simulink library "GFo_Lib_old"  (R2017a)
settings: Solver=VariableStepAuto  StartTime=0.0  StopTime=10.0  RelTol=1e-3
undefined symbols (not defined in the file or in its folder): C_line, Time_Step, VSC01_id0
undefined symbols (not defined in the file): VSC01_Cf, VSC01_Lf, VSC01_Rf
libraries: powerlib x25, Control_Lib x12, simulink x7, powerlib_meascontrol x2
(part 1 of 2)
settings Model: Creator=Frederic_Colas  LastModifiedBy=Frederic_Colas

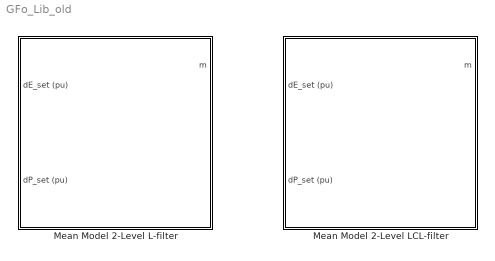
== system GFo_Lib_old ==
  Mean Model 2-Level L-filter : Subsystem  mask(VSC){fn=50, Sn=1000e6, Pn=1000e6, Udcn=640e3, Un1=320e3, Un2=400e3, Rt_pu=0.005, Lt_pu=0.15, Lm_pu=500, Rm_pu=500, Tr_PLL=10e-3, Val_Freq_Support=on, R_percent=4, Rv=0.009, W_TVR=60, I_thresh_pu=1, DX_DR=5, Kp_Rvi_pu=0.676, gainpopup=3, wc1=31.4159, mp1=0.0043, wc2=33.3, mp2=0.0033, wc3=2.5, mp3=0.04, T1=0.1210, T2=0.022, LFpopup=PQ, P0=0.5, Q0=0, V0=1, Theta0=0.57242}
      mask prompts: fn "Nominal Frequency (Hz)"; Sn "Nominal Apparent Power (VA)"; Pn "Nominal Power (W)"; Udcn "Nominal DC Voltage (V)"; Un1 "VSC side Nominal Ph-Ph Voltage (V)"; Un2 "Grid side Nominal Ph-Ph Voltage (V)"; Rt_pu "R (pu)"; Lt_pu "L (pu)"; Lm_pu "Rm (pu)"; Rm_pu "Lm (pu)"; Tr_PLL "Time response (s)"; Val_Freq_Support "Frequency Support"; R_percent "Droop Gain (%)"; Rv "Damping Resistance (Rv)"; W_TVR "Dr filter"; I_thresh_pu "Current Threshold (pu)"; Kp_Rvi_pu "Kp_Rvi"; gainpopup "Strategy"; wc1 "wc"; mp1 "mp"; wc2 "wc"; mp2 "mp"; wc3 "wc"; mp3 "mp"; P0 "Initial Active Power (pu)"; Q0 "Initial Reactive Power (pu)"; V0 "Initial Voltage (pu)"; Theta0 "Initial Angle (°)"
      mask init:
      | % Update Name of LF bus for internal purpose
      |     NameStr = [get_param(gcb,'Name')];% '_LF'];
      |     set_param([gcb '/Load Flow Bus'],'ID',NameStr);    
      |     
      | % Base values
      |     fb = fn;
      |     Pb = Pn;
      |     cos_phi_n = Pn/Sn;
      |     Sb = Pb/cos_phi_n;
      |     Vn1 = Un1/sqrt(3);
      |     Vb1 = Vn1;
      |     Vn2 = Un2/sqrt(3);
      |     Vb2 = Vn2;
      |     Ib1 = Sb / 3*Vb1;
      |     Ib2 = Sb / (3*Vb2);
      |     wb = 2*pi*fb;
      |   
      | % PLL derivation of the parameters
      |     wn_PLL=5/Tr_PLL;
      |     zeta_PLL = 1;
      |     Kp_PLL_pu = 2*zeta_PLL*wn_PLL/wb;
      |     Ki_PLL_pu = wn_PLL^2/wb;
      |     
      | % Set the chosen strategy
      |     Chosen_Strategy = gainpopup;
      |     
      | % Set the frequency droop gain
      |     R = R_percent / 100;
      | 
      | % Compute Initial Voltage of VSC 
      | %   from steady-state output transformer model and Loadflow result
      |     
      |     %Initialize correctly the LoadFlow bus parameters connected to PCC
      |     VLF = V0;
      |     ThetaLF = Theta0;
      |     if (LFpopup == 'PQ')
      |         VLF = 1;
      |         ThetaLF = 0;
      |     elseif (LFpopup == 'PV')
      |         VLF = V0;
      |         ThetaLF = 0;        
      |     end
      |     set_param([gcb '/Load Flow Bus'],'Vref',num2str(VLF),'Vangle',num2str(ThetaLF));
      |     
      |     R1_pu = Rt_pu/2;
      |     L1_pu = Lt_pu/2;
      |     R2_pu = Rt_pu/2;
      |     L2_pu = Lt_pu/2;
      |     X1_pu = L1_pu;
      |     X2_pu = L2_pu;
      |     Xm_pu = Lm_pu;
      |     
      |     Zm_pu = 1/(1/Rm_pu+1/(1i*Xm_pu));
      | 
      |     S0=P0+1i*Q0;
      |     I2 = conj(S0)/(V0);
      | 
      |     Vm = (R2_pu+1i*X2_pu)*I2 + V0;
      |     Im = Vm/Zm_pu;
      | 
      |     I1 = I2 + Im;
      |     V1 = (R1_pu+1i*X1_pu) * I1 + Vm;
      | 
      |     Vvsc0 = abs(V1);
      |     Theta_vsc0 = angle(V1) * 180/pi+Theta0;
      |     
      |     Va0 = Vvsc0*sqrt(2)*Vb1*sin(Theta_vsc0*pi/180);
      |     Vb0 = Vvsc0*sqrt(2)*Vb1*sin(Theta_vsc0*pi/180-2*pi/3);
      |     Vc0 = Vvsc0*sqrt(2)*Vb1*sin(Theta_vsc0*pi/180+2*pi/3);
      |     
      | % Generate string to display LF results on Mask
      |     %str_tmp = fprintf("Vvsc0 = %d, Theta_vsc0 = %d°",Vvsc0,Theta_vsc0);
      |     mo = get_param(gcb,'MaskObject');
      |     mo.getDialogControl('LF_vsc_str').Prompt = ['V0 = ', num2str(Vvsc0),' pu, Angle = ', num2str(Theta_vsc0),'°'];
      |     mo.getDialogControl('LF_pcc_str').Prompt = ['V0 = ', num2str(V0),' pu, Angle = ', num2str(Theta0),'°'];
      |     mo.getDialogControl('LF_pcc_Power_str').Prompt = ['P0 = ', num2str(P0),' pu, Q0 = ', num2str(Q0),' pu'];
      |     %set_param([gcb],'LF_str',str_tmp);
      settings: OpenFcn=|
      | NameStr = get_param(gcb,'Name');
      | open_system(gcbh, 'Mask');
      | 
      | h2AllOpenDlgs = DAStudio.ToolRoot.getOpenDialogs;
      | 
      | for i=1:length(h2AllOpenDlgs)
      |     try
      |          %disp(h2AllOpenDlgs(i).getSource.getBlock.Name);
      |         Dialog_block_name = h2AllOpenDlgs(i).getSource.getBlock.Name;
      |          %strcmp(Dialog_block_name, NameStr),
      |         if (strcmp(h2AllOpenDlgs(i).getSource.getBlock.Name, NameStr))
      |             iPos = h2AllOpenDlgs(i).position;
      |             h2AllOpenDlgs(i).position = [iPos(1)   iPos(2)   iPos(3)*1.4   iPos(4)];
      |         end
      |     end
      | end
      mask TypeOptions gainpopup: 1 | 2 | 3
      mask Callback gainpopup:
      | % Get the mask parameter values. This is a cell
      | %   array of character vectors.
      | maskStr = get_param(gcb,'gainpopup');
      | p=Simulink.Mask.get(gcb);
      | 
      | % The pop-up menu is the first mask parameter.
      | %   Check the value selected in the pop-up
      | if strcmp(maskStr,'1'),
      | 
      |     % Set the visibility of both parameters on when
      |     %   User-defined is selected in the pop-up.
      |     p.getDialogControl('Param_Strat_1').Visible='on';
      |     p.getDialogControl('Param_Strat_2').Visible='off';
      |     p.getDialogControl('Param_Strat_3').Visible='off';
      | 
      | elseif strcmp(maskStr,'2'),
      | 
      |     % Set the visibility of both parameters on when
      |     %   User-defined is selected in the pop-up.
      |     p.getDialogControl('Param_Strat_1').Visible='off';
      |     p.getDialogControl('Param_Strat_2').Visible='on';
      |     p.getDialogControl('Param_Strat_3').Visible='off';
      | 
      |     % Turn off the visibility of the Value field
      |     %   when User-defined is not selected.
      | else
      | 
      |     % Set the visibility of both parameters on when
      |     %   User-defined is selected in the pop-up.
      |     p.getDialogControl('Param_Strat_1').Visible='off';
      |     p.getDialogControl('Param_Strat_2').Visible='off';
      |     p.getDialogControl('Param_Strat_3').Visible='on';
      | 
      | end
      mask TypeOptions LFpopup: Swing | PQ | PV
      mask Callback LFpopup:
      | % Get the mask parameter values. This is a cell
      | %   array of character vectors.
      | maskStr = get_param(gcb,'LFpopup');
      | p=Simulink.Mask.get(gcb);
      | 
      | % The pop-up menu is the first mask parameter.
      | %   Check the value selected in the pop-up
      | if strcmp(maskStr,'Swing'),
      | 
      |     % Set the visibility of both parameters on when
      |     %   User-defined is selected in the pop-up.
      |     p.getParameter('P0').Visible='off';
      |     p.getParameter('Q0').Visible='off';
      |     p.getParameter('V0').Visible='on';
      |     p.getParameter('Theta0').Visible='on';
      |     set_param([gcb '/Source_For_LF'],'BusType','swing');
      | 
      | elseif strcmp(maskStr,'PQ'),
      | 
      |     % Set the visibility of both parameters on when
      |     %   User-defined is selected in the pop-up.
      |     p.getParameter('P0').Visible='on';
      |     p.getParameter('Q0').Visible='on';
      |     p.getParameter('V0').Visible='off';
      |     p.getParameter('Theta0').Visible='off';
      |     set_param([gcb '/Source_For_LF'],'BusType','PQ');
      | 
      |     % Turn off the visibility of the Value field
      |     %   when User-defined is not selected.
      | else
      | 
      |     % Set the visibility of both parameters on when
      |     %   User-defined is selected in the pop-up.
      |     p.getParameter('P0').Visible='on';
      |     p.getParameter('Q0').Visible='off';
      |     p.getParameter('V0').Visible='on';
      |     p.getParameter('Theta0').Visible='off';
      |     set_param([gcb '/Source_For_LF'],'BusType','PV');
      | 
      | end
      mask DialogControl Title_Strat_1 Prompt: Strategy 1
      mask DialogControl Title_Strat_2 Prompt: Strategy 2
      mask DialogControl Title_Strat_3 Prompt: Strategy 3
      mask DialogControl Control4 Prompt: Initial Operating Point
      mask DialogControl Container24 Prompt: VSC side
      mask DialogControl LF_vsc_str Prompt: V0 = 1.0055 pu, Angle = 4.8589°
      mask DialogControl Container25 Prompt: PCC
      mask DialogControl UpdateLoadflow Prompt: Update Loadflow
      mask DialogControl UpdateLoadflow Callback: LoadFlow_VSC
      mask Display:
      | disp('L-Filter');
      | port_label('input',1,'dE_set (pu)');
      | port_label('input',2,'dP_set (pu)');
      | port_label('output',1,'m');
      | port_label('rconn',1,'A');
      | port_label('rconn',2,'B');
      | port_label('rconn',3,'C');
  Mean Model 2-Level LCL-filter : Subsystem  mask(VSC){fn=50, Sn=1000e6, Pn=1000e6, Udcn=640e3, Un1=320e3, Un2=400e3, Rt_pu=0.005, Lt_pu=0.15, Rm_pu=500, Lm_pu=500, Lf_pu=0.15, Rf_pu=0.005, Cf_pu=0.066, Tr_PLL=10e-3, Val_Freq_Support=on, Val_gamma=on, R_percent=4, Rv=0.009, W_TVR=60, I_thresh_pu=1, DX_DR=5, Kp_Rvi_pu=0.676, gainpopup=3, wc1=31.4159, mp1=0.0043, wc2=33.3, mp2=0.0033, wc3=2.5, mp3=0.04, T1=0.1210, T2=0.022, LFpopup=PV, P0=0.1, Q0=0, V0=1, Theta0=13.5501, innercontrol=1, Kp_i=0.73, Ki_i=1.19, Kp_v=0.52, Ki_v=1.16, Kffv=1, Kffi=1, I_max=1.25}
      mask prompts: fn "Nominal Frequency (Hz)"; Sn "Nominal Apparent Power (VA)"; Pn "Nominal Power (W)"; Udcn "Nominal DC Voltage (V)"; Un1 "VSC side Nominal Ph-Ph Voltage (V)"; Un2 "Grid side Nominal Ph-Ph Voltage (V)"; Rt_pu "R (pu)"; Lt_pu "L (pu)"; Rm_pu "Rm (pu)"; Lm_pu "Lm (pu)"; Lf_pu "Lf (pu)"; Rf_pu "Rf (pu)"; Cf_pu "Cf (pu)"; Tr_PLL "Time response (s)"; Val_Freq_Support "Frequency Support"; Val_gamma "gamma activation"; R_percent "Droop Gain (%)"; Rv "Damping Resistance (Rv)"; W_TVR "Dr filter"; I_thresh_pu "Current Threshold (pu)"; Kp_Rvi_pu "Kp_Rvi"; gainpopup "Strategy"; wc1 "wc"; mp1 "mp"; wc2 "wc"; mp2 "mp"; wc3 "wc"; mp3 "mp"; P0 "Initial Active Power (pu)"; Q0 "Initial Reactive Power (pu)"; V0 "Initial Voltage (pu)"; Theta0 "Initial Angle (°)"; innercontrol "Strategy"
      mask init:
      | % Update Name of LF bus for internal purpose
      |     NameStr = [get_param(gcb,'Name')];% '_LF'];
      |     set_param([gcb '/Load Flow Bus'],'ID',NameStr);
      |     %disp(NameStr);
      | 
      | % Base values
      |     % 1 = VSC side
      |     % 2 = grid side
      |     fb = fn;
      |     Pb = Pn;
      |     cos_phi_n = Pn/Sn;
      |     Sb = Pb/cos_phi_n;
      |     Vn1 = Un1/sqrt(3);
      |     Vb1 = Vn1;
      |     Vn2 = Un2/sqrt(3);
      |     Vb2 = Vn2;
      |     Ib1 = Sb / (3*Vb1);
      |     Ib2 = Sb / (3*Vb2);
      |     Zb = (3*Vb1^2)/Sb;
      |     wb = 2*pi*fb;  wb_pu=1;
      |     Lb = Zb/wb;
      |     Cb = 1/(Zb*wb);
      |   
      | % PLL derivation of the parameters
      |     wn_PLL=5/Tr_PLL;
      |     zeta_PLL = 1;
      |     Kp_PLL_pu = 2*zeta_PLL*wn_PLL/wb;
      |     Ki_PLL_pu = wn_PLL^2/wb;
      |     
      | % Set the chosen strategy
      |     Chosen_Strategy = gainpopup;
      |     
      | % Set the frequency droop gain
      |     R = R_percent/100;
      | 
      | % Compute Initial Voltage of VSC 
      | %   from steady-state output transformer model and Loadflow result
      |     
      |     %Initialize correctly the LoadFlow bus parameters connected to PCC
      |     VLF = V0;
      |     ThetaLF = Theta0;
      |     if (LFpopup == 'PQ')
      |         VLF = 1;
      |         ThetaLF = 0;
      |     elseif (LFpopup == 'PV')
      |         VLF = V0;
      |         ThetaLF = 0;        
      |     end
      |     set_param([gcb '/Load Flow Bus'],'Vref',num2str(VLF),'Vangle',num2str(ThetaLF));
      | 
      |     % steady-state model of output transformer
      |     Rf_pu = Rt_pu;
      |     R1_pu = Rt_pu/2;
      |     L1_pu = Lt_pu/2;
      |     R2_pu = Rt_pu/2;
      |     L2_pu = Lt_pu/2;
      |     X1_pu = L1_pu;
      |     X2_pu = L2_pu;
      |     Xm_pu = Lm_pu;
      |     wb_pu = 1;
      |     
      |     Zm_pu = 1/(1/Rm_pu+1/(1i*Xm_pu));
      |     S0=P0+1i*Q0;
      |     I2 = conj(S0)/(V0);
      |     Vm = (R2_pu+1i*X2_pu)*I2 + V0;
      |     Im = Vm/Zm_pu;
      |     I1 = I2 + Im;
      |     V1 = (R1_pu+1i*X1_pu) * I1 + Vm;
      |     
      |     Eg0 = abs(V1); % compute initial Eg value
      |     Theta_m0 = angle(V1) * 180/pi+Theta0;
      |     
      |     %Steady-state model of LC Filter
      |     Is = I1 + 1i*Cf_pu*V1;
      |     Theta_Is = angle(Is) * 180/pi+Theta0;
      |     Vm = (1i*Lf_pu+Rf_pu)*Is+ V1;  %  
      |     
      | % Generate string to display LF results on Mask
      |     %str_tmp = fprintf("Vvsc0 = %d, Theta_vsc0 = %d°",Vvsc0,Theta_vsc0);
      |     mo = get_param(gcb,'MaskObject');
      |     mo.getDialogControl('LF_pcc_str').Prompt = ['V0 = ', num2str(V0),' pu, Angle = ', num2str(Theta0),'°'];
      |     mo.getDialogControl('LF_pcc_Power_str').Prompt = ['P0 = ', num2str(P0),' pu, Q0 = ', num2str(Q0),' pu'];
      |     %set_param([gcb],'LF_str',str_tmp);
      |  %GRD00_Theta0 = Theta0;
      |  % Initial current and voltage states calculation 
      |  
      | % Given Setpoint in PV bus
      |  
      | Vg0_d=V0*cos(Theta0*pi/180-Theta_m0*pi/180);
      | Vg0_q=V0*sin(Theta0*pi/180-Theta_m0*pi/180);
      | Vg0_dq = [Vg0_d ;Vg0_q; 0];
      |  
      | % Initial state of AC grid current : Ig0dq
      | 
      | Theta_I2 = angle(I2) * 180/pi + Theta0;
      | Ig0_d = abs(I2)*cos(Theta_I2*pi/180-Theta_m0*pi/180);
      | Ig0_q = abs(I2)*sin(Theta_I2*pi/180-Theta_m0*pi/180);
      | Ig0_dq = [Ig0_d; Ig0_q; 0];
      |  
      | % Initial state of capacitor voltage : eg0dq
      | 
      | Eg0_d = Eg0;
      | Eg0_q = 0;
      | Eg0_dq = [Eg0; 0; 0];
      |  
      | % Initial state of VSC Current : Is0dq
      | 
      | Is0_d = abs(Is) * cos(Theta_Is*pi/180-Theta_m0*pi/180);
      | Is0_q = abs(Is) * sin(Theta_Is*pi/180-Theta_m0*pi/180);
      | Is0_dq = [Is0_d; Is0_q; 0];
      | 
      | % Initial state of Modulation Voltage : Vm0dq
      | 
      | Vvsc0 = abs(Vm);
      | Theta_vsc0 = angle(Vm)*180/pi + Theta0;
      | Vm0_d = Vvsc0 * cos(Theta_vsc0*pi/180-Theta_m0*pi/180);
      | Vm0_q = Vvsc0 * sin(Theta_vsc0*pi/180-Theta_m0*pi/180);
      |  
      | Va0 = sqrt(2)*Vb1*Vvsc0*sin(Theta_vsc0*pi/180);
      | Vb0 = sqrt(2)*Vb1*Vvsc0*sin(Theta_vsc0*pi/180-2*pi/3);
      | Vc0 = sqrt(2)*Vb1*Vvsc0*sin(Theta_vsc0*pi/180+2*pi/3);
      | Vabc0 = [Va0 Vb0 Vc0];
      |  
      | mo.getDialogControl('LF_vsc_str').Prompt = ['V0 = ', num2str(Eg0),' pu, Angle = ', num2str(Theta_m0),'°'];
      settings: OpenFcn=|
      | NameStr = get_param(gcb,'Name');
      | open_system(gcbh, 'Mask');
      | 
      | h2AllOpenDlgs = DAStudio.ToolRoot.getOpenDialogs;
      | 
      | for i=1:length(h2AllOpenDlgs)
      |     try
      |          %disp(h2AllOpenDlgs(i).getSource.getBlock.Name);
      |         Dialog_block_name = h2AllOpenDlgs(i).getSource.getBlock.Name;
      |          %strcmp(Dialog_block_name, NameStr),
      |         if (strcmp(h2AllOpenDlgs(i).getSource.getBlock.Name, NameStr))
      |             iPos = h2AllOpenDlgs(i).position;
      |             h2AllOpenDlgs(i).position = [iPos(1)   iPos(2)   iPos(3)*1.6   iPos(4)];
      |         end
      |     end
      | end
      mask TypeOptions gainpopup: 1 | 2 | 3
      mask Callback gainpopup:
      | % Get the mask parameter values. This is a cell
      | %   array of character vectors.
      | maskStr = get_param(gcb,'gainpopup');
      | p=Simulink.Mask.get(gcb);
      | 
      | % The pop-up menu is the first mask parameter.
      | %   Check the value selected in the pop-up
      | if strcmp(maskStr,'1'),
      | 
      |     % Set the visibility of both parameters on when
      |     %   User-defined is selected in the pop-up.
      |     p.getDialogControl('Param_Strat_1').Visible='on';
      |     p.getDialogControl('Param_Strat_2').Visible='off';
      |     p.getDialogControl('Param_Strat_3').Visible='off';
      | 
      | 
      | elseif strcmp(maskStr,'2'),
      | 
      |     % Set the visibility of both parameters on when
      |     %   User-defined is selected in the pop-up.
      |     p.getDialogControl('Param_Strat_1').Visible='off';
      |     p.getDialogControl('Param_Strat_2').Visible='on';
      |     p.getDialogControl('Param_Strat_3').Visible='off';
      | 
      | 
      |     % Turn off the visibility of the Value field
      |     %   when User-defined is not selected.
      | elseif strcmp(maskStr,'3'),
      | 
      |     % Set the visibility of both parameters on when
      |     %   User-defined is selected in the pop-up.
      |     p.getDialogControl('Param_Strat_1').Visible='off';
      |     p.getDialogControl('Param_Strat_2').Visible='off';
      |     p.getDialogControl('Param_Strat_3').Visible='on';
      | 
      | else
      | 
      |     % Set the visibility of both parameters on when
      |     %   User-defined is selected in the pop-up.
      |     p.getDialogControl('Param_Strat_1').Visible='off';
      |     p.getDialogControl('Param_Strat_2').Visible='off';
      |     p.getDialogControl('Param_Strat_3').Visible='off';
      | 
      | end
      mask TypeOptions LFpopup: Swing | PQ | PV
      mask Callback LFpopup:
      | % Get the mask parameter values. This is a cell
      | %   array of character vectors.
      | maskStr = get_param(gcb,'LFpopup');
      | p=Simulink.Mask.get(gcb);
      | 
      | % The pop-up menu is the first mask parameter.
      | %   Check the value selected in the pop-up
      | if strcmp(maskStr,'Swing'),
      | 
      |     % Set the visibility of both parameters on when
      |     %   User-defined is selected in the pop-up.
      |     p.getParameter('P0').Visible='off';
      |     p.getParameter('Q0').Visible='off';
      |     p.getParameter('V0').Visible='on';
      |     p.getParameter('Theta0').Visible='on';
      |     set_param([gcb '/Source_For_LF'],'BusType','swing');
      | 
      | elseif strcmp(maskStr,'PQ'),
      | 
      |     % Set the visibility of both parameters on when
      |     %   User-defined is selected in the pop-up.
      |     p.getParameter('P0').Visible='on';
      |     p.getParameter('Q0').Visible='on';
      |     %p.getParameter('V0').Value='1';
      |     %set_param(gcb,'V0','1');
      |     p.getParameter('V0').Visible='off';
      |     p.getParameter('Theta0').Visible='off';
      |     set_param([gcb '/Source_For_LF'],'BusType','PQ');
      | 
      |     % Turn off the visibility of the Value field
      |     %   when User-defined is not selected.
      | else
      | 
      |     % Set the visibility of both parameters on when
      |     %   User-defined is selected in the pop-up.
      |     p.getParameter('P0').Visible='on';
      |     p.getParameter('Q0').Visible='off';
      |     p.getParameter('V0').Visible='on';
      |     p.getParameter('Theta0').Visible='off';
      |     set_param([gcb '/Source_For_LF'],'BusType','PV');
      | 
      | end
      mask TypeOptions innercontrol: 1
      mask Callback innercontrol:
      | % Get the mask parameter values. This is a cell
      | %   array of character vectors.
      | maskStr = get_param(gcb,'innercontrol');
      | p=Simulink.Mask.get(gcb);
      | 
      | % The pop-up menu is the first mask parameter.
      | %   Check the value selected in the pop-up
      | if strcmp(maskStr,'1'),
      | 
      |     % Set the visibility of both parameters on when
      |     %   User-defined is selected in the pop-up.
      |     p.getDialogControl('Param_Strat_11').Visible='on';
      | 
      | 
      | else
      | 
      |     % Set the visibility of both parameters on when
      |     %   User-defined is selected in the pop-up.
      |     p.getDialogControl('Param_Strat_11').Visible='on';
      | 
      | end
      mask DialogControl Title_Strat_1 Prompt: Strategy 1
      mask DialogControl Title_Strat_2 Prompt: Strategy 2
      mask DialogControl Title_Strat_3 Prompt: Strategy 3
      mask DialogControl Control4 Prompt: Initial Operating Point
      mask DialogControl Container24 Prompt: VSC side
      mask DialogControl LF_vsc_str Prompt: V0 = 1.0008 pu, Angle = 14.4173°
      mask DialogControl Container25 Prompt: PCC
      mask DialogControl UpdateLoadflow Prompt: Update Loadflow
      mask DialogControl UpdateLoadflow Callback: LoadFlow_VSC
      mask DialogControl Title_Strat_11 Prompt: Cascaded_control
      mask Display:
      | disp('LCL-Filter');
      | port_label('input',1,'dE_set (pu)');
      | port_label('input',2,'dP_set (pu)');
      | port_label('output',1,'m');
      | port_label('rconn',1,'A');
      | port_label('rconn',2,'B');
      | port_label('rconn',3,'C');

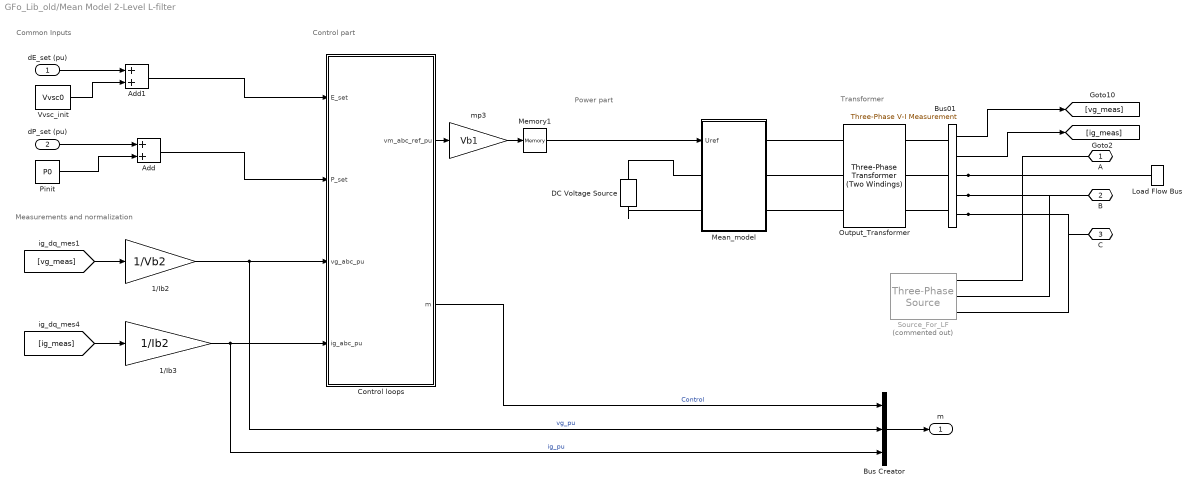
== system GFo_Lib_old/Mean Model 2-Level L-filter ==
  note: Control part
  note: Measurements and normalization
  note: Power part
  note: Common Inputs
  note: Transformer
  dE_set (pu) : Inport
  dP_set (pu) : Inport  Port=2
  1/Ib2 : Gain  Gain=1/Vb2
  1/Ib3 : Gain  Gain=1/Ib2
  Add : Sum
  Add1 : Sum
  Bus Creator : BusCreator  Inputs=3
  Bus01 : powerlib/Measurements/Three-Phase V-I Measurement  VoltageMeasurement=phase-to-ground  SetLabelV=off  LabelV=Vabc  Vpu=off  VpuLL=off  CurrentMeasurement=yes  SetLabelI=off  LabelI=Iabc  Ipu=off  Pbase=100e6  Vbase=500e3  OutputType=Complex  PhasorSimulation=off  PSBequivalent=0
  Control loops : Subsystem
  DC Voltage Source : powerlib/Electrical Sources/DC Voltage Source  Amplitude=Udcn  Measurements=Voltage
  Load Flow Bus : powerlib/Measurements/Load Flow Bus  LConnTagsString=a  Phases=single  Connectors=on one side  ID=Mean Model 2-Level L-filter  Vbase=Un2  Vref=1  Vangle=0.57242  VLF=1.001  VLFb=1  VLFc=1  angleLF=0.5724  angleLFb=0  angleLFc=0
      settings: SourceProductName=Simscape Power Systems
  Mean_model : Subsystem
  Memory1 : Memory  X0=[Va0 Vb0 Vc0]
  Output_Transformer : powerlib/Elements/Three-Phase Transformer (Two Windings)  Winding1Connection=Yg  Winding2Connection=Yg  CoreType=Three single-phase transformers  SetSaturation=off  Hysteresis=off  DataFile='hysteresis'  SetInitialFlux=off  Measurements=None  UNITS=pu  NominalPower=[Sn , fb]  Winding1=[Un1 , Rt_pu/2 , Lt_pu/2]  Winding2=[Un2 , Rt_pu/2 , Lt_pu/2]  Rm=Rm_pu  Lm=Lm_pu  L0=0.5  Saturation=[ 0,0 ; 0.0024,1.2 ; 1.0,1.52 ]  InitialFluxes=[ 0.8 , -0.8 , 0.7 ]  MoreParameters=off  BreakLoop=off  DataType=off  TransfoNumber=1
  Pinit : Constant  Value=P0
  Source_For_LF : powerlib/Electrical Sources/Three-Phase Source  Commented=on  InternalConnection=Yg  VoltagePhases=off  Voltage=Un2  PhaseAngle=0  Voltage_phases=[25e3 25e3 25e3]/sqrt(3)  PhaseAngles_phases=[0 -120 +120]  Frequency=fb  NonIdealSource=off  SpecifyImpedance=off  Resistance=0  Inductance=0  ShortCircuitLevel=100e6  BaseVoltage=Un  XRratio=7  BusType=PQ  Pref=P0*Sb  Qref=Q0*Sb  Prefabc=[10e3, 10e3, 10e3]  Qrefabc=[0, 0, 0]  Qmin=-inf  Qmax=inf
  Vvsc_init : Constant  Value=Vvsc0
  mp3 : Gain  Gain=Vb1
  A : PMIOPort  Port=1  Side=Right
  B : PMIOPort  Port=2  Side=Right
  C : PMIOPort  Port=3  Side=Right
  m : Outport
  wires:
  [ig_meas] -> 1/Ib3/1
  Bus01/2 -> [ig_meas]
  dE_set (pu)/1 -> Add1/1
  Bus01/1 -> [vg_meas]
  Vvsc_init/1 -> Add1/2
  Pinit/1 -> Add/2
  dP_set (pu)/1 -> Add/1
  Memory1/1 -> Mean_model/1(Uref)
  Add1/1 -> Control loops/1(E_set)
  Control loops/1(vm_abc_ref_pu) -> mp3/1
  [vg_meas] -> 1/Ib2/1
  Bus Creator/1 -> m/1
  1/Ib2/1 -> Control loops/3(vg_abc_pu), Bus Creator/2  "vg_pu"
  1/Ib3/1 -> Control loops/4(ig_abc_pu), Bus Creator/3  "ig_pu"
  mp3/1 -> Memory1/1
  Control loops/2(m) -> Bus Creator/1  "Control"
  Add/1 -> Control loops/2(P_set)
  connections:
  Bus01/RConn3 -- C/RConn1 -- Source_For_LF/RConn3
  Bus01/RConn1 -- A/RConn1 -- Load Flow Bus/LConn1 -- Source_For_LF/RConn1
  Mean_model/RConn3 -- Output_Transformer/LConn3
  Mean_model/RConn2 -- Output_Transformer/LConn2
  Mean_model/RConn1 -- Output_Transformer/LConn1
  Bus01/RConn2 -- B/RConn1 -- Source_For_LF/RConn2
  Output_Transformer/RConn3 -- Bus01/LConn3
  DC Voltage Source/RConn1 -- Mean_model/LConn1
  Output_Transformer/RConn2 -- Bus01/LConn2
  Output_Transformer/RConn1 -- Bus01/LConn1
  DC Voltage Source/LConn1 -- Mean_model/LConn2

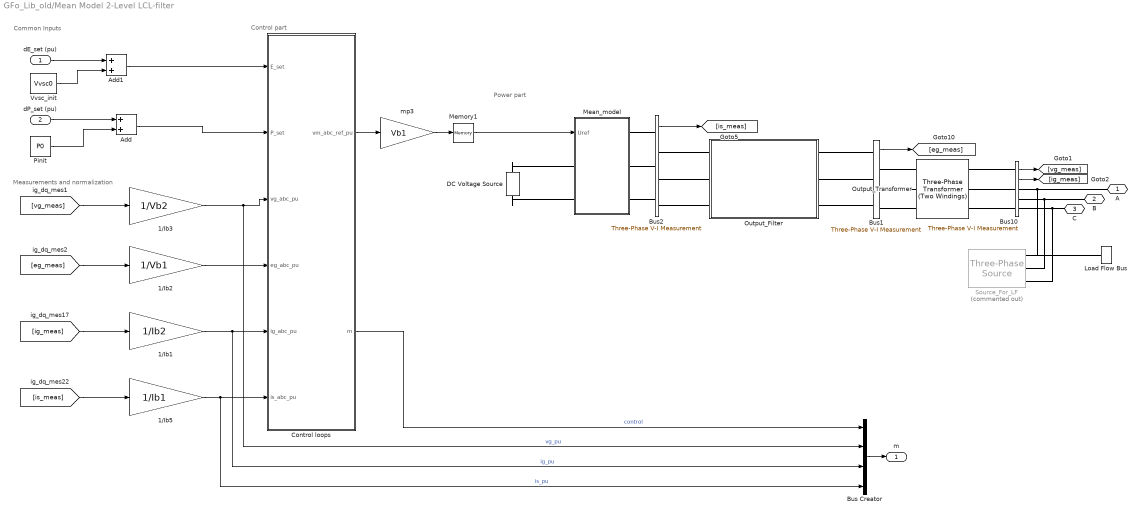
== system GFo_Lib_old/Mean Model 2-Level LCL-filter ==
  note: Control part
  note: Measurements and normalization
  note: Power part
  note: Common Inputs
  dE_set (pu) : Inport
  dP_set (pu) : Inport  Port=2
  1/Ib1 : Gain  Gain=1/Ib2
  1/Ib2 : Gain  Gain=1/Vb1
  1/Ib3 : Gain  Gain=1/Vb2
  1/Ib5 : Gain  Gain=1/Ib1
  Add : Sum
  Add1 : Sum
  Bus Creator : BusCreator  Inputs=4
  Bus1 : powerlib/Measurements/Three-Phase V-I Measurement  VoltageMeasurement=phase-to-ground  SetLabelV=off  LabelV=Vabc  Vpu=off  VpuLL=off  CurrentMeasurement=no  SetLabelI=off  LabelI=Iabc  Ipu=off  Pbase=100e6  Vbase=500e3  OutputType=Complex  PhasorSimulation=off  PSBequivalent=0
  Bus10 : powerlib/Measurements/Three-Phase V-I Measurement  VoltageMeasurement=phase-to-ground  SetLabelV=off  LabelV=Vabc  Vpu=off  VpuLL=off  CurrentMeasurement=yes  SetLabelI=off  LabelI=Iabc  Ipu=off  Pbase=100e6  Vbase=500e3  OutputType=Complex  PhasorSimulation=off  PSBequivalent=0
  Bus2 : powerlib/Measurements/Three-Phase V-I Measurement  VoltageMeasurement=no  SetLabelV=off  LabelV=Vabc  Vpu=off  VpuLL=off  CurrentMeasurement=yes  SetLabelI=off  LabelI=Iabc  Ipu=off  Pbase=100e6  Vbase=500e3  OutputType=Complex  PhasorSimulation=off  PSBequivalent=0
  Control loops : Subsystem
  DC Voltage Source : powerlib/Electrical Sources/DC Voltage Source  Amplitude=Udcn  Measurements=Voltage
  Load Flow Bus : powerlib/Measurements/Load Flow Bus  LConnTagsString=a  Phases=single  Connectors=on one side  ID=Mean Model 2-Level LCL-filter  Vbase=Un2  Vref=1  Vangle=13.5501  VLF=0.9956  VLFb=1  VLFc=1  angleLF=13.55  angleLFb=0  angleLFc=0
      settings: SourceProductName=Simscape Power Systems
  Mean_model : Subsystem
  Memory1 : Memory  X0=[Va0 Vb0 Vc0]
  Output_Filter : Subsystem  mask{Lf=VSC01_Lf, Rf=VSC01_Rf, Cf=VSC01_Cf}
      mask prompts: Lf "Filter inductance [H]"; Rf "Filter resistance [R]"; Cf "Filter capacitance [F]"
  Output_Transformer : powerlib/Elements/Three-Phase Transformer (Two Windings)  Winding1Connection=Yg  Winding2Connection=Yg  CoreType=Three single-phase transformers  SetSaturation=off  Hysteresis=off  DataFile='hysteresis'  SetInitialFlux=off  Measurements=None  UNITS=pu  NominalPower=[Sn , fb]  Winding1=[Un1 , Rt_pu/2 , Lt_pu/2]  Winding2=[Un2 , Rt_pu/2 , Lt_pu/2]  Rm=Rm_pu  Lm=Lm_pu  L0=0.5  Saturation=[ 0,0 ; 0.0024,1.2 ; 1.0,1.52 ]  InitialFluxes=[-1.0109960716468 0.506091473811006 0.504904597835851]  MoreParameters=off  BreakLoop=off  DataType=off  TransfoNumber=1
  Pinit : Constant  Value=P0
  Source_For_LF : powerlib/Electrical Sources/Three-Phase Source  Commented=on  InternalConnection=Yg  VoltagePhases=off  Voltage=Un2*V0  PhaseAngle=Theta0  Voltage_phases=[25e3 25e3 25e3]/sqrt(3)  PhaseAngles_phases=[0 -120 +120]  Frequency=fb  NonIdealSource=off  SpecifyImpedance=off  Resistance=0  Inductance=0  ShortCircuitLevel=100e6  BaseVoltage=Un  XRratio=7  BusType=PV  Pref=P0*Sb  Qref=Q0*Sb  Prefabc=[10e3, 10e3, 10e3]  Qrefabc=[0, 0, 0]  Qmin=-inf  Qmax=inf
  Vvsc_init : Constant  Value=Vvsc0
  mp3 : Gain  Gain=Vb1
  A : PMIOPort  Port=1  Side=Right
  B : PMIOPort  Port=2  Side=Right
  C : PMIOPort  Port=3  Side=Right
  m : Outport
  wires:
  Add/1 -> Control loops/2(P_set)
  dE_set (pu)/1 -> Add1/1
  Bus1/1 -> [eg_meas]
  Add1/1 -> Control loops/1(E_set)
  Vvsc_init/1 -> Add1/2
  Pinit/1 -> Add/2
  dP_set (pu)/1 -> Add/1
  Bus10/1 -> [vg_meas]
  Bus2/1 -> [is_meas]
  mp3/1 -> Memory1/1
  Bus10/2 -> [ig_meas]
  1/Ib1/1 -> Control loops/5(ig_abc_pu), Bus Creator/3  "ig_pu"
  1/Ib3/1 -> Bus Creator/2, Control loops/3(vg_abc_pu)  "vg_pu"
  Control loops/2(m) -> Bus Creator/1  "control"
  Bus Creator/1 -> m/1
  1/Ib2/1 -> Control loops/4(eg_abc_pu)
  1/Ib5/1 -> Control loops/6(is_abc_pu), Bus Creator/4  "is_pu"
  Control loops/1(vm_abc_ref_pu) -> mp3/1
  Memory1/1 -> Mean_model/1(Uref)
  [vg_meas] -> 1/Ib3/1
  [eg_meas] -> 1/Ib2/1
  [ig_meas] -> 1/Ib1/1
  [is_meas] -> 1/Ib5/1
  connections:
  DC Voltage Source/RConn1 -- Mean_model/LConn1
  DC Voltage Source/LConn1 -- Mean_model/LConn2
  Bus1/LConn1 -- Output_Filter/RConn1
  Bus1/LConn2 -- Output_Filter/RConn2
  Bus1/LConn3 -- Output_Filter/RConn3
  Output_Transformer/LConn1 -- Bus1/RConn1
  Bus1/RConn2 -- Output_Transformer/LConn2
  Bus1/RConn3 -- Output_Transformer/LConn3
  Bus10/LConn1 -- Output_Transformer/RConn1
  Bus10/LConn2 -- Output_Transformer/RConn2
  Bus10/LConn3 -- Output_Transformer/RConn3
  C/RConn1 -- Source_For_LF/RConn3 -- Bus10/RConn3
  B/RConn1 -- Source_For_LF/RConn2 -- Bus10/RConn2
  A/RConn1 -- Load Flow Bus/LConn1 -- Source_For_LF/RConn1 -- Bus10/RConn1
  Bus2/LConn1 -- Mean_model/RConn1
  Bus2/LConn2 -- Mean_model/RConn2
  Bus2/LConn3 -- Mean_model/RConn3
  Bus2/RConn1 -- Output_Filter/LConn1
  Bus2/RConn2 -- Output_Filter/LConn2
  Bus2/RConn3 -- Output_Filter/LConn3

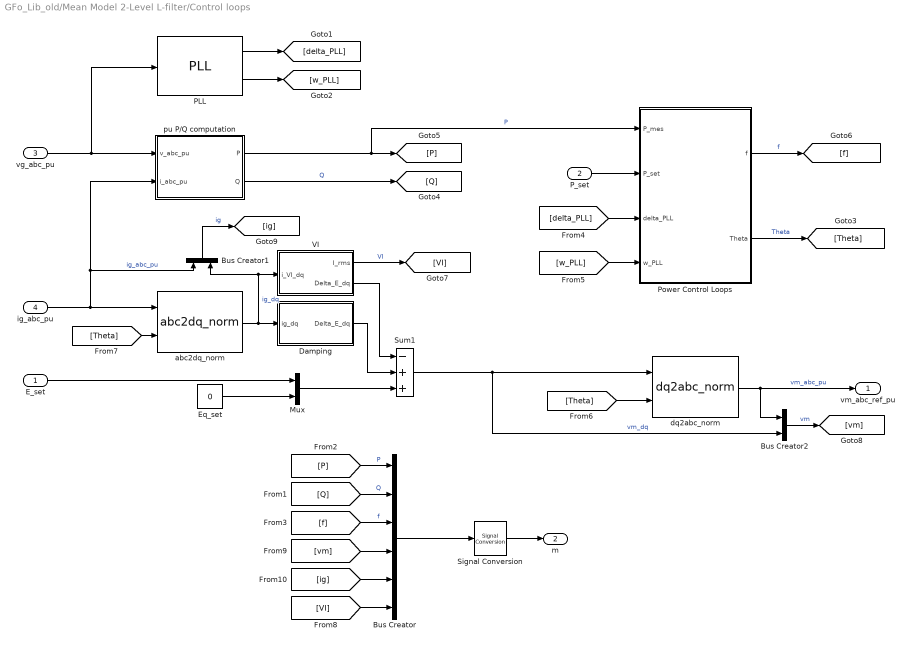
== system GFo_Lib_old/Mean Model 2-Level L-filter/Control loops ==
  E_set : Inport
  P_set : Inport  Port=2
  vg_abc_pu : Inport  Port=3
  ig_abc_pu : Inport  Port=4
  " pu P/Q computation" : Subsystem  DialogController=POWERSYS.PowerSysDialog
  Bus Creator : BusCreator  Inputs=6
  Bus Creator1 : BusCreator  Inputs=2
  Bus Creator2 : BusCreator  Inputs=2
  Damping : Subsystem
  Eq_set : Constant  Value=0
  Mux : Mux  Inputs=2
  PLL : Control_Lib/PLL  fb=fb  Tr_PLL=Tr_PLL*1000  zeta_PLL=1  Theta0=Theta0
      settings: SourceProductName=VSC4SPS
  Power Control Loops : Subsystem
  Signal Conversion : SignalConversion  OverrideOpt=off
  Sum1 : Sum  Inputs=-++
  VI : Subsystem
  abc2dq_norm : Control_Lib/abc2dq_norm
      settings: SourceProductName=VSC4SPS
  dq2abc_norm : Control_Lib/dq2abc_norm
      settings: SourceProductName=VSC4SPS
  vm_abc_ref_pu : Outport
  m : Outport  Port=2
  wires:
  Signal Conversion/1 -> m/1
  [P] -> Bus Creator/1  "P"
  [Q] -> Bus Creator/2  "Q"
  [f] -> Bus Creator/3  "f"
  dq2abc_norm/1 -> vm_abc_ref_pu/1, Bus Creator2/1  "vm_abc_pu"
  E_set/1 -> Mux/1
  " pu P/Q computation"/2(Q) -> [Q]  "Q"
  Sum1/1 -> dq2abc_norm/1, Bus Creator2/2  "vm_dq"
  [delta_PLL] -> Power Control Loops/3(delta_PLL)
  P_set/1 -> Power Control Loops/2(P_set)
  [w_PLL] -> Power Control Loops/4(w_PLL)
  Power Control Loops/1(f) -> [f]  "f"
  vg_abc_pu/1 -> PLL/1, " pu P/Q computation"/1(v_abc_pu)
  " pu P/Q computation"/1(P) -> Power Control Loops/1(P_mes), [P]  "P"
  ig_abc_pu/1 -> abc2dq_norm/1, Bus Creator1/1, " pu P/Q computation"/2(i_abc_pu)  "ig_abc_pu"
  abc2dq_norm/1 -> Damping/1(ig_dq), VI/1(i_VI_dq), Bus Creator1/2  "ig_dq"
  Power Control Loops/2(Theta) -> [Theta]  "Theta"
  [Theta] -> dq2abc_norm/2
  [Theta] -> abc2dq_norm/2
  VI/2(Delta_E_dq) -> Sum1/1
  Damping/1("Delta_E_dq ") -> Sum1/2
  VI/1(I_rms) -> [VI]  "VI"
  Mux/1 -> Sum1/3
  Eq_set/1 -> Mux/2
  Bus Creator2/1 -> [vm]  "vm"
  [vm] -> Bus Creator/4
  [VI] -> Bus Creator/6
  Bus Creator/1 -> Signal Conversion/1
  Bus Creator1/1 -> [ig]  "ig"
  [ig] -> Bus Creator/5
  PLL/1 -> [delta_PLL]
  PLL/2 -> [w_PLL]

== system GFo_Lib_old/Mean Model 2-Level L-filter/Mean_model ==
  Uref : Inport
  NOT1 : Logic  Operator=NOT  IconShape=distinctive  AllPortsSameDT=off  OutDataTypeStr=boolean
  Step1 : Step  Time=Time_Step  SampleTime=Time_Step
  Terminator : Terminator
  Three-Phase Breaker1 : powerlib/Elements/Three-Phase Breaker  InitialState=closed  SwitchA=on  SwitchB=on  SwitchC=on  SwitchTimes="[4/60  10/60]"  External=on  BreakerResistance=0.001  SnubberResistance=1e6  SnubberCapacitance=inf  Measurements=None
  Three-Phase Breaker2 : powerlib/Elements/Three-Phase Breaker  InitialState=open  SwitchA=on  SwitchB=on  SwitchC=on  SwitchTimes="[4/60  10/60]"  External=on  BreakerResistance=0.001  SnubberResistance=1e6  SnubberCapacitance=inf  Measurements=None
  Three-Phase Source : powerlib/Electrical Sources/Three-Phase Source  InternalConnection=Yg  VoltagePhases=off  Voltage=Vvsc0*Un1  PhaseAngle=Theta_vsc0  Voltage_phases=[25e3 25e3 25e3]/sqrt(3)  PhaseAngles_phases=[0 -120 +120]  Frequency=fb  NonIdealSource=off  SpecifyImpedance=off  Resistance=0  Inductance=0  ShortCircuitLevel=100e6  BaseVoltage=VSC01_Un1  XRratio=7  BusType=swing  Pref=0.3  Qref=0  Prefabc=[10e3, 10e3, 10e3]  Qrefabc=[0, 0, 0]  Qmin=-Inf  Qmax=Inf
  Universal Bridge : powerlib/Power Electronics/Universal Bridge  Arms=3  SnubberResistance=1e5  SnubberCapacitance=inf  Device=Average-model based VSC  Ron=1e-3  Lon=0  ForwardVoltages="[  0  0  ]"  ForwardVoltage=0  GTOparameters=[ 10e-6 , 20e-6 ]  IGBTparameters=[ 1e-6 , 2e-6 ]  Measurements=None  Measurements_2=None  converterType=Rectifier
  Vdc : powerlib/Measurements/Voltage Measurement  PhasorSimulation=off  OutputType=Complex  PSBequivalent=0
  mp3 : Gain  Gain=2/Udcn
  PhA : PMIOPort  Port=1  Side=Right
  PhB : PMIOPort  Port=2  Side=Right
  PhC : PMIOPort  Port=3  Side=Right
  Vdc+ : PMIOPort  Port=4  Side=Left
  Vdc- : PMIOPort  Port=5  Side=Left
  wires:
  Vdc/1 -> Terminator/1
  Uref/1 -> mp3/1
  mp3/1 -> Universal Bridge/1
  Step1/1 -> Three-Phase Breaker2/1, NOT1/1
  NOT1/1 -> Three-Phase Breaker1/1
  connections:
  Vdc-/RConn1 -- Universal Bridge/RConn2 -- Vdc/LConn2
  Vdc+/RConn1 -- Universal Bridge/RConn1 -- Vdc/LConn1
  Three-Phase Source/RConn3 -- Three-Phase Breaker1/RConn3
  Three-Phase Source/RConn2 -- Three-Phase Breaker1/RConn2
  Three-Phase Source/RConn1 -- Three-Phase Breaker1/RConn1
  Three-Phase Breaker2/RConn3 -- Universal Bridge/LConn3
  Three-Phase Breaker2/RConn2 -- Universal Bridge/LConn2
  Three-Phase Breaker2/RConn1 -- Universal Bridge/LConn1
  PhC/RConn1 -- Three-Phase Breaker1/LConn3 -- Three-Phase Breaker2/LConn3
  PhB/RConn1 -- Three-Phase Breaker1/LConn2 -- Three-Phase Breaker2/LConn2
  PhA/RConn1 -- Three-Phase Breaker1/LConn1 -- Three-Phase Breaker2/LConn1

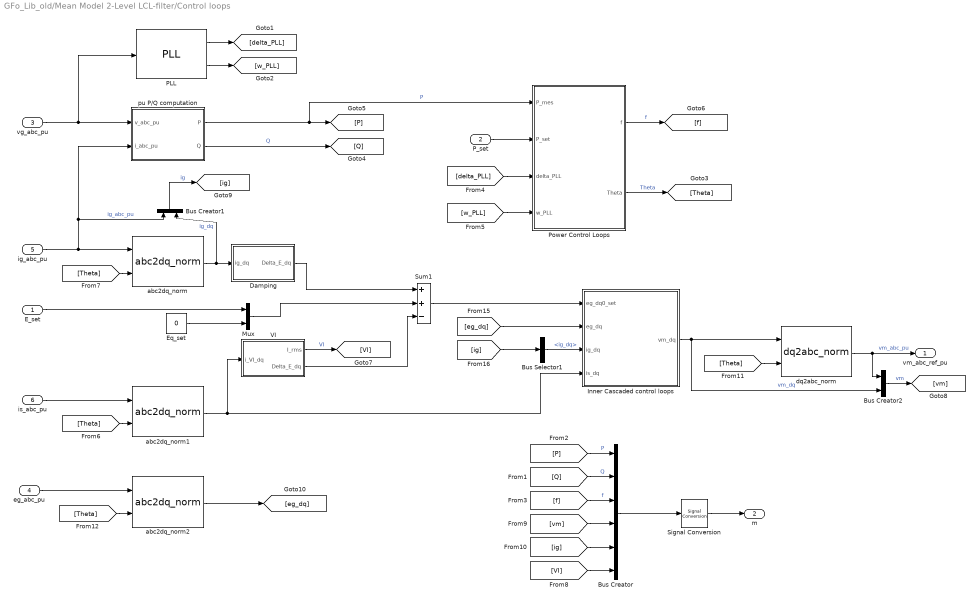
== system GFo_Lib_old/Mean Model 2-Level LCL-filter/Control loops ==
  E_set : Inport
  P_set : Inport  Port=2
  vg_abc_pu : Inport  Port=3
  eg_abc_pu : Inport  Port=4
  ig_abc_pu : Inport  Port=5
  is_abc_pu : Inport  Port=6
  " pu P/Q computation" : Subsystem  DialogController=POWERSYS.PowerSysDialog
  Bus Creator : BusCreator  Inputs=6
  Bus Creator1 : BusCreator  Inputs=2
  Bus Creator2 : BusCreator  Inputs=2
  Bus Selector1 : BusSelector  OutputSignals=ig_dq
  Damping : Subsystem
  Eq_set : Constant  Value=0
  Inner Cascaded control loops : Subsystem
  Mux : Mux  Inputs=2
  PLL : Control_Lib/PLL  fb=fb  Tr_PLL=Tr_PLL*1000  zeta_PLL=1  Theta0=Theta0
      settings: SourceProductName=VSC4SPS
  Power Control Loops : Subsystem
  Signal Conversion : SignalConversion  OverrideOpt=off
  Sum1 : Sum  Inputs=++-
  VI : Subsystem
  abc2dq_norm : Control_Lib/abc2dq_norm
      settings: SourceProductName=VSC4SPS
  abc2dq_norm1 : Control_Lib/abc2dq_norm
      settings: SourceProductName=VSC4SPS
  abc2dq_norm2 : Control_Lib/abc2dq_norm
      settings: SourceProductName=VSC4SPS
  dq2abc_norm : Control_Lib/dq2abc_norm
      settings: SourceProductName=VSC4SPS
  vm_abc_ref_pu : Outport
  m : Outport  Port=2
  wires:
  Signal Conversion/1 -> m/1
  [P] -> Bus Creator/1  "P"
  [Q] -> Bus Creator/2  "Q"
  [f] -> Bus Creator/3  "f"
  E_set/1 -> Mux/1
  " pu P/Q computation"/2(Q) -> [Q]  "Q"
  [delta_PLL] -> Power Control Loops/3(delta_PLL)
  P_set/1 -> Power Control Loops/2(P_set)
  [w_PLL] -> Power Control Loops/4(w_PLL)
  Power Control Loops/1(f) -> [f]  "f"
  " pu P/Q computation"/1(P) -> Power Control Loops/1(P_mes), [P]  "P"
  ig_abc_pu/1 -> abc2dq_norm/1, Bus Creator1/1, " pu P/Q computation"/2(i_abc_pu)  "ig_abc_pu"
  abc2dq_norm/1 -> Damping/1(ig_dq), Bus Creator1/2  "ig_dq"
  Power Control Loops/2(Theta) -> [Theta]  "Theta"
  [Theta] -> abc2dq_norm/2
  VI/2(Delta_E_dq) -> Sum1/3
  Damping/1("Delta_E_dq ") -> Sum1/1
  VI/1(I_rms) -> [VI]  "VI"
  Mux/1 -> Sum1/2
  Eq_set/1 -> Mux/2
  [vm] -> Bus Creator/4
  [VI] -> Bus Creator/6
  Bus Creator/1 -> Signal Conversion/1
  Bus Creator1/1 -> [ig]  "ig"
  [ig] -> Bus Creator/5
  [Theta] -> abc2dq_norm1/2
  vg_abc_pu/1 -> PLL/1, " pu P/Q computation"/1(v_abc_pu)
  abc2dq_norm1/1 -> Inner Cascaded control loops/4(is_dq), VI/1(i_VI_dq)
  [Theta] -> abc2dq_norm2/2
  abc2dq_norm2/1 -> [eg_dq]
  is_abc_pu/1 -> abc2dq_norm1/1
  eg_abc_pu/1 -> abc2dq_norm2/1
  [eg_dq] -> Inner Cascaded control loops/2(eg_dq)
  Inner Cascaded control loops/1(vm_dq) -> dq2abc_norm/1, Bus Creator2/2  "vm_dq"
  dq2abc_norm/1 -> Bus Creator2/1, vm_abc_ref_pu/1  "vm_abc_pu"
  [Theta] -> dq2abc_norm/2
  Bus Creator2/1 -> [vm]  "vm"
  Bus Selector1/1 -> Inner Cascaded control loops/3(ig_dq)  "<ig_dq>"
  [ig] -> Bus Selector1/1
  Sum1/1 -> Inner Cascaded control loops/1(eg_dq0_set)
  PLL/1 -> [delta_PLL]
  PLL/2 -> [w_PLL]

== system GFo_Lib_old/Mean Model 2-Level LCL-filter/Mean_model ==
  Uref : Inport
  NOT1 : Logic  Operator=NOT  IconShape=distinctive  AllPortsSameDT=off  OutDataTypeStr=boolean
  Step1 : Step  Time=Time_Step  SampleTime=Time_Step
  Terminator : Terminator
  Three-Phase Breaker1 : powerlib/Elements/Three-Phase Breaker  InitialState=closed  SwitchA=on  SwitchB=on  SwitchC=on  SwitchTimes="[4/60  10/60]"  External=on  BreakerResistance=0.001  SnubberResistance=1e6  SnubberCapacitance=inf  Measurements=None
  Three-Phase Breaker2 : powerlib/Elements/Three-Phase Breaker  InitialState=open  SwitchA=on  SwitchB=on  SwitchC=on  SwitchTimes="[4/60  10/60]"  External=on  BreakerResistance=0.001  SnubberResistance=1e6  SnubberCapacitance=inf  Measurements=None
  Three-Phase Source : powerlib/Electrical Sources/Three-Phase Source  InternalConnection=Yg  VoltagePhases=off  Voltage=Vvsc0*Un1  PhaseAngle=Theta_vsc0  Voltage_phases=[25e3 25e3 25e3]/sqrt(3)  PhaseAngles_phases=[0 -120 +120]  Frequency=fb  NonIdealSource=off  SpecifyImpedance=off  Resistance=0  Inductance=0  ShortCircuitLevel=100e6  BaseVoltage=VSC01_Un1  XRratio=7  BusType=swing  Pref=0.3  Qref=0  Prefabc=[10e3, 10e3, 10e3]  Qrefabc=[0, 0, 0]  Qmin=-Inf  Qmax=Inf
  Universal Bridge : powerlib/Power Electronics/Universal Bridge  Arms=3  SnubberResistance=1e5  SnubberCapacitance=inf  Device=Average-model based VSC  Ron=1e-3  Lon=0  ForwardVoltages="[  0  0  ]"  ForwardVoltage=0  GTOparameters=[ 10e-6 , 20e-6 ]  IGBTparameters=[ 1e-6 , 2e-6 ]  Measurements=None  Measurements_2=None  converterType=Rectifier
  Vdc : powerlib/Measurements/Voltage Measurement  PhasorSimulation=off  OutputType=Complex  PSBequivalent=0
  mp3 : Gain  Gain=2/Udcn
  PhA : PMIOPort  Port=1  Side=Right
  PhB : PMIOPort  Port=2  Side=Right
  PhC : PMIOPort  Port=3  Side=Right
  Vdc+ : PMIOPort  Port=4  Side=Left
  Vdc- : PMIOPort  Port=5  Side=Left
  wires:
  Vdc/1 -> Terminator/1
  Uref/1 -> mp3/1
  mp3/1 -> Universal Bridge/1
  Step1/1 -> Three-Phase Breaker2/1, NOT1/1
  NOT1/1 -> Three-Phase Breaker1/1
  connections:
  Vdc-/RConn1 -- Universal Bridge/RConn2 -- Vdc/LConn2
  Vdc+/RConn1 -- Universal Bridge/RConn1 -- Vdc/LConn1
  Three-Phase Source/RConn3 -- Three-Phase Breaker1/RConn3
  Three-Phase Source/RConn2 -- Three-Phase Breaker1/RConn2
  Three-Phase Source/RConn1 -- Three-Phase Breaker1/RConn1
  Three-Phase Breaker2/RConn3 -- Universal Bridge/LConn3
  Three-Phase Breaker2/RConn2 -- Universal Bridge/LConn2
  Three-Phase Breaker2/RConn1 -- Universal Bridge/LConn1
  PhC/RConn1 -- Three-Phase Breaker1/LConn3 -- Three-Phase Breaker2/LConn3
  PhB/RConn1 -- Three-Phase Breaker1/LConn2 -- Three-Phase Breaker2/LConn2
  PhA/RConn1 -- Three-Phase Breaker1/LConn1 -- Three-Phase Breaker2/LConn1

== system GFo_Lib_old/Mean Model 2-Level LCL-filter/Output_Filter ==
  Filter capacitance : powerlib/Elements/Three-Phase Series RLC Branch  LConnTagsString=A|B|C  RConnTagsString=A|B|C  BranchType=C  Resistance=0  Inductance=C_line(1)  Capacitance=Cf_pu*Cb  Measurements=None
  Filter inductance : powerlib/Elements/Three-Phase Series RLC Branch  LConnTagsString=A|B|C  RConnTagsString=A|B|C  BranchType=RL  Resistance=Rf_pu*Zb  Inductance=Lf_pu*Lb  Capacitance=1e-6  Measurements=None
  Ground : powerlib/Elements/Ground  LConnTagsString=a
  A : PMIOPort  Port=1  Side=Left
  a : PMIOPort  Port=2  Side=Right
  B : PMIOPort  Port=3  Side=Left
  b : PMIOPort  Port=4  Side=Right
  C : PMIOPort  Port=5  Side=Left
  c : PMIOPort  Port=6  Side=Right
  connections:
  Filter inductance/RConn1 -- Filter capacitance/LConn1 -- a/RConn1
  Filter inductance/RConn3 -- Filter capacitance/LConn3 -- c/RConn1
  Filter inductance/LConn2 -- B/RConn1
  Filter inductance/LConn3 -- C/RConn1
  Filter inductance/LConn1 -- A/RConn1
  Filter inductance/RConn2 -- Filter capacitance/LConn2 -- b/RConn1
  Filter capacitance/RConn2 -- Filter capacitance/RConn3 -- Filter capacitance/RConn1 -- Ground/LConn1

== system GFo_Lib_old/Mean Model 2-Level L-filter/Control loops/ pu P//Q computation ==
  v_abc_pu : Inport  PortDimensions=3
  i_abc_pu : Inport  Port=2  PortDimensions=3
  Demux : Demux  Outputs=3
  Mux : Mux  Inputs=3
  Product1 : Product  SaturateOnIntegerOverflow=on  InputSameDT=on  OutDataTypeStr=Inherit: Same as first input
  Product3 : Product  SaturateOnIntegerOverflow=on  InputSameDT=on  OutDataTypeStr=Inherit: Same as first input
  Sum : Sum  Inputs=+-  SaturateOnIntegerOverflow=on  InputSameDT=on  OutDataTypeStr=Inherit: Same as first input
  Sum1 : Sum  Inputs=1  SaturateOnIntegerOverflow=on  InputSameDT=on  OutDataTypeStr=Inherit: Same as first input
  Sum4 : Sum  Inputs=1  SaturateOnIntegerOverflow=on  InputSameDT=on  OutDataTypeStr=Inherit: Same as first input
  Sum5 : Sum  Inputs=+-  SaturateOnIntegerOverflow=on  InputSameDT=on  OutDataTypeStr=Inherit: Same as first input
  Sum6 : Sum  Inputs=+-  SaturateOnIntegerOverflow=on  InputSameDT=on  OutDataTypeStr=Inherit: Same as first input
  pu->V : Gain  Gain=1/sqrt(3)  SaturateOnIntegerOverflow=on  OutDataTypeStr=Inherit: Same as input  ParamDataTypeStr=Inherit: Same as input
  pu->V1 : Gain  Gain=1/3  SaturateOnIntegerOverflow=on  OutDataTypeStr=Inherit: Same as input  ParamDataTypeStr=Inherit: Same as input
  pu->V2 : Gain  Gain=1/3  SaturateOnIntegerOverflow=on  OutDataTypeStr=Inherit: Same as input  ParamDataTypeStr=Inherit: Same as input
  P : Outport
  Q : Outport  Port=2
  wires:
  pu->V/1 -> pu->V2/1  "Q"
  Mux/1 -> Product3/1
  Sum6/1 -> Mux/2
  Sum5/1 -> Mux/1
  Sum/1 -> Mux/3
  Demux/3 -> Sum6/1, Sum5/2
  Demux/2 -> Sum5/1, Sum/2
  Demux/1 -> Sum6/2, Sum/1
  Sum4/1 -> pu->V1/1
  i_abc_pu/1 -> Product3/2, Product1/2
  v_abc_pu/1 -> Demux/1, Product1/1
  Product1/1 -> Sum4/1
  Product3/1 -> Sum1/1
  Sum1/1 -> pu->V/1
  pu->V1/1 -> P/1
  pu->V2/1 -> Q/1

== system GFo_Lib_old/Mean Model 2-Level L-filter/Control loops/Damping ==
  ig_dq : Inport
  Filter w_LF : Subsystem
      mask Display: disp('\omega_{LF} / (s + \omega_{LF})','texmode','on')
  Sum5 : Sum  Inputs=|+-
  nq1 : Gain  Gain=Rv
  "Delta_E_dq " : Outport
  wires:
  ig_dq/1 -> nq1/1
  Sum5/1 -> "Delta_E_dq "/1
  Filter w_LF/1(s) -> Sum5/1
  nq1/1 -> Sum5/2, Filter w_LF/1(e)

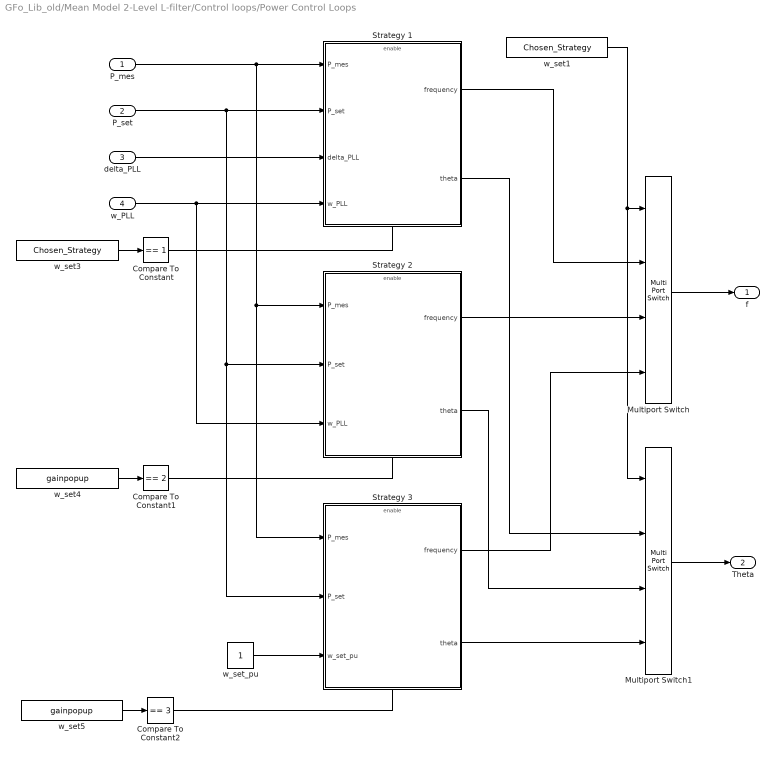
== system GFo_Lib_old/Mean Model 2-Level L-filter/Control loops/Power Control Loops ==
  P_mes : Inport
  P_set : Inport  Port=2
  delta_PLL : Inport  Port=3
  w_PLL : Inport  Port=4
  Compare To Constant : simulink/Logic and Bit Operations/Compare To Constant  relop===  const=1  OutDataTypeStr=boolean
  Compare To Constant1 : simulink/Logic and Bit Operations/Compare To Constant  relop===  const=2  OutDataTypeStr=boolean
  Compare To Constant2 : simulink/Logic and Bit Operations/Compare To Constant  relop===  const=3  OutDataTypeStr=boolean
  Multiport Switch : MultiPortSwitch
  Multiport Switch1 : MultiPortSwitch
  Strategy 1 : Subsystem
  Strategy 2 : Subsystem
  Strategy 3 : Subsystem
  w_set1 : Constant  Value=Chosen_Strategy
  w_set3 : Constant  Value=Chosen_Strategy
  w_set4 : Constant  Value=gainpopup
  w_set5 : Constant  Value=gainpopup
  w_set_pu : Constant
  f : Outport
  Theta : Outport  Port=2
  wires:
  P_mes/1 -> Strategy 3/1(P_mes), Strategy 2/1(P_mes), Strategy 1/1(P_mes)
  P_set/1 -> Strategy 2/2(P_set), Strategy 3/2(P_set), Strategy 1/2(P_set)
  delta_PLL/1 -> Strategy 1/3(delta_PLL)
  w_PLL/1 -> Strategy 2/3(w_PLL), Strategy 1/4(w_PLL)
  w_set_pu/1 -> Strategy 3/3(w_set_pu)
  Strategy 3/2(theta) -> Multiport Switch1/4
  Strategy 3/1(frequency) -> Multiport Switch/4
  Strategy 2/1(frequency) -> Multiport Switch/3
  w_set1/1 -> Multiport Switch1/1, Multiport Switch/1
  Strategy 2/2(theta) -> Multiport Switch1/3
  Multiport Switch1/1 -> Theta/1
  Strategy 1/2(theta) -> Multiport Switch1/2
  Multiport Switch/1 -> f/1
  Strategy 1/1(frequency) -> Multiport Switch/2
  w_set3/1 -> Compare To Constant/1
  w_set4/1 -> Compare To Constant1/1
  w_set5/1 -> Compare To Constant2/1
  Compare To Constant/1 -> Strategy 1/Enable
  Compare To Constant1/1 -> Strategy 2/Enable
  Compare To Constant2/1 -> Strategy 3/Enable

== system GFo_Lib_old/Mean Model 2-Level L-filter/Control loops/VI ==
  note: VI
  note: VI triggering and threshold computation
  i_VI_dq : Inport
  Bus Creator : BusCreator  Inputs=1
  Demux1 : Demux  Outputs=2
  Gain5 : Gain  Gain=DX_DR
  Gain6 : Gain  Gain=Kp_Rvi_pu
  Gain9 : Gain  Gain=DX_DR
  I_thresh : Constant  Value=I_thresh_pu
  Mux2 : Mux  Inputs=2
  Saturation : Saturate  UpperLimit=inf  LowerLimit=0
  Sum1 : Sum  Inputs=-+|
  Sum7 : Sum  Inputs=|+-
  Sum8 : Sum  Inputs=++|
  dq to phasor : Subsystem
  product{,1..3} (4 alike) : Product  SaturateOnIntegerOverflow=on  RndMeth=Zero  InputSameDT=on  OutDataTypeStr=Inherit: Same as first input
  I_rms : Outport
  Delta_E_dq : Outport  Port=2
  wires:
  i_VI_dq/1 -> Demux1/1, dq to phasor/1(dq_mes)
  Sum8/1 -> Mux2/2
  Sum7/1 -> Mux2/1
  product2/1 -> Sum8/2
  Gain9/1 -> Sum8/1
  Gain5/1 -> Sum7/2
  product1/1 -> Sum7/1
  Demux1/2 -> product3/1, product2/1  "igq"
  Demux1/1 -> product/2, product1/1  "igd"
  product/1 -> Gain9/1
  product3/1 -> Gain5/1
  Gain6/1 -> product2/2, product1/2, product/1, product3/2
  Mux2/1 -> Delta_E_dq/1
  I_thresh/1 -> Sum1/1
  Saturation/1 -> Gain6/1
  dq to phasor/1(rms) -> Bus Creator/1, Sum1/2  "I_rms"
  Sum1/1 -> Saturation/1
  Bus Creator/1 -> I_rms/1

== system GFo_Lib_old/Mean Model 2-Level LCL-filter/Control loops/ pu P//Q computation ==
  v_abc_pu : Inport  PortDimensions=3
  i_abc_pu : Inport  Port=2  PortDimensions=3
  Demux : Demux  Outputs=3
  Mux : Mux  Inputs=3
  Product1 : Product  SaturateOnIntegerOverflow=on  InputSameDT=on  OutDataTypeStr=Inherit: Same as first input
  Product3 : Product  SaturateOnIntegerOverflow=on  InputSameDT=on  OutDataTypeStr=Inherit: Same as first input
  Sum : Sum  Inputs=+-  SaturateOnIntegerOverflow=on  InputSameDT=on  OutDataTypeStr=Inherit: Same as first input
  Sum1 : Sum  Inputs=1  SaturateOnIntegerOverflow=on  InputSameDT=on  OutDataTypeStr=Inherit: Same as first input
  Sum4 : Sum  Inputs=1  SaturateOnIntegerOverflow=on  InputSameDT=on  OutDataTypeStr=Inherit: Same as first input
  Sum5 : Sum  Inputs=+-  SaturateOnIntegerOverflow=on  InputSameDT=on  OutDataTypeStr=Inherit: Same as first input
  Sum6 : Sum  Inputs=+-  SaturateOnIntegerOverflow=on  InputSameDT=on  OutDataTypeStr=Inherit: Same as first input
  pu->V : Gain  Gain=1/sqrt(3)  SaturateOnIntegerOverflow=on  OutDataTypeStr=Inherit: Same as input  ParamDataTypeStr=Inherit: Same as input
  pu->V1 : Gain  Gain=1/3  SaturateOnIntegerOverflow=on  OutDataTypeStr=Inherit: Same as input  ParamDataTypeStr=Inherit: Same as input
  pu->V2 : Gain  Gain=1/3  SaturateOnIntegerOverflow=on  OutDataTypeStr=Inherit: Same as input  ParamDataTypeStr=Inherit: Same as input
  P : Outport
  Q : Outport  Port=2
  wires:
  pu->V/1 -> pu->V2/1  "Q"
  Mux/1 -> Product3/1
  Sum6/1 -> Mux/2
  Sum5/1 -> Mux/1
  Sum/1 -> Mux/3
  Demux/3 -> Sum6/1, Sum5/2
  Demux/2 -> Sum5/1, Sum/2
  Demux/1 -> Sum6/2, Sum/1
  Sum4/1 -> pu->V1/1
  i_abc_pu/1 -> Product3/2, Product1/2
  v_abc_pu/1 -> Demux/1, Product1/1
  Product1/1 -> Sum4/1
  Product3/1 -> Sum1/1
  Sum1/1 -> pu->V/1
  pu->V1/1 -> P/1
  pu->V2/1 -> Q/1

== system GFo_Lib_old/Mean Model 2-Level LCL-filter/Control loops/Damping ==
  ig_dq : Inport
  Filter w_LF : Subsystem
      mask Display: disp('\omega_{LF} / (s + \omega_{LF})','texmode','on')
  Sum5 : Sum  Inputs=|+-
  nq1 : Gain  Gain=Rv
  "Delta_E_dq " : Outport
  wires:
  ig_dq/1 -> nq1/1
  Sum5/1 -> "Delta_E_dq "/1
  Filter w_LF/1(s) -> Sum5/1
  nq1/1 -> Sum5/2, Filter w_LF/1(e)

== system GFo_Lib_old/Mean Model 2-Level LCL-filter/Control loops/Inner Cascaded control loops ==
  eg_dq0_set : Inport
  eg_dq : Inport  Port=2
  ig_dq : Inport  Port=3
  is_dq : Inport  Port=4
  Amplitude : Subsystem
  Compare To Constant : simulink/Logic and Bit Operations/Compare To Constant  relop=<=  const=I_max  OutDataTypeStr=boolean
  Current PI control : Subsystem
  Memory : Memory  X0=1
  Voltage PI control : Subsystem
  w_pu : Constant
  vm_dq : Outport
  wires:
  Amplitude/2(cond) -> Compare To Constant/1
  eg_dq0_set/1 -> Voltage PI control/2(Eg_dq0_ref)
  Voltage PI control/1(Is_dq0_ref) -> Amplitude/1(is_unsat)
  Amplitude/1(is_sat) -> Current PI control/3(Is_dq0_ref)
  w_pu/1 -> Current PI control/4(w), Voltage PI control/4(w)
  Current PI control/1(Vm_dq0_ref) -> vm_dq/1
  is_dq/1 -> Current PI control/1(Is_dq0)
  eg_dq/1 -> Current PI control/2(Eg_dq0), Voltage PI control/1(Eg_dq0)
  ig_dq/1 -> Voltage PI control/3(Ig_dq0)
  Compare To Constant/1 -> Memory/1
  Memory/1 -> Voltage PI control/5(block integ)
